simulink model "new_lv_trygenerator_mode1"  (Simulink 7.1)
settings: Solver=ode3  StartTime=0.0  StopTime=1000  FixedStep=0.01  RelTol=1e-3
values from neighbouring files (symbols this model uses):
  Jem = 90    [lv_cankaofile.m]    (also in lv_demofile.m = 97.5; lv_demofile1.m = 97.5; lv_demofile2.m = 97.5; lv_demofile3.m = 97.5)
  Jwt = 9e7    (= 90000000)    [lv_cankaofile.m]    (also in lv_demofile.m = 3275300; lv_demofile1.m = 3275300; lv_demofile2.m = 3275300; lv_demofile3.m = 3275300)
  K = 83    [lv_cankaofile.m]    (also in lv_demofile.m; lv_demofile1.m = 75.76; lv_demofile2.m; lv_demofile3.m = 75.76)
  R = 40    [lv_cankaofile.m]    (also in lv_demofile.m = 38.5; lv_demofile1.m = 38.75; lv_demofile2.m = 38.5; lv_demofile3.m = 38.5)
  ro_air = 1.225    [lv_cankaofile.m]    (also in lv_demofile.m = 1.2236; lv_demofile1.m; lv_demofile2.m = 1.2236; lv_demofile3.m)
libraries: simulink x1, DRlib x1
settings Model: Creator=lv  LastModifiedBy=lv

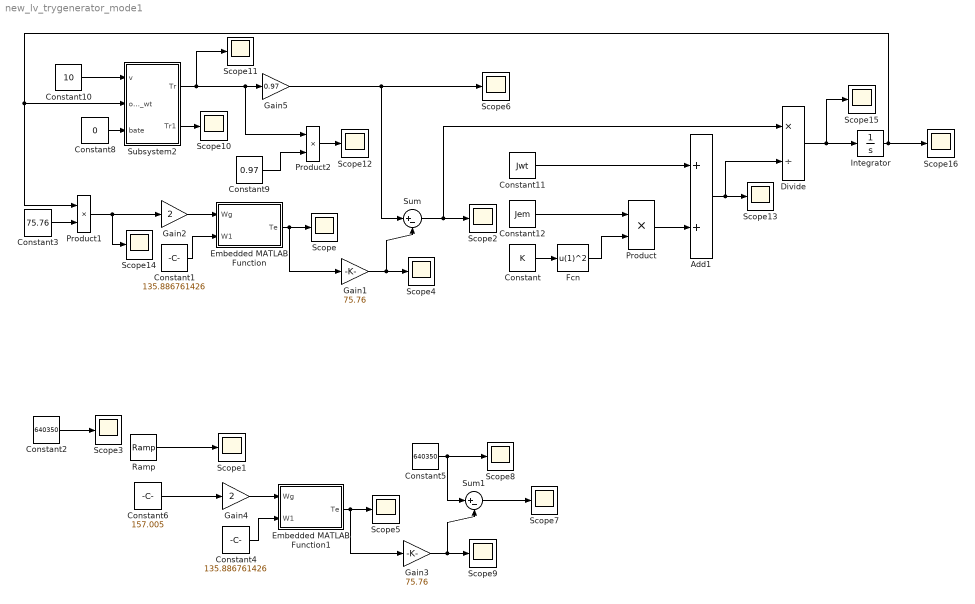
== system new_lv_trygenerator_mode1 ==
  Add1 : Sum  OutDataType=sfix(16)  OutScaling=2^-10
  Constant : Constant  Value=K  OutDataType=sfix(16)  OutScaling=2^0
  Constant1 : Constant  Value=135.886761426  OutDataType=sfix(16)  OutScaling=2^0
  Constant10 : Constant  Value=10  VectorParams1D=off  OutDataType=sfix(16)  OutScaling=2^0
  Constant11 : Constant  Value=Jwt  OutDataType=sfix(16)  OutScaling=2^0
  Constant12 : Constant  Value=Jem  OutDataType=sfix(16)  OutScaling=2^0
  Constant2 : Constant  Value=640350  OutDataType=sfix(16)  OutScaling=2^0
  Constant3 : Constant  Value=75.76  OutDataType=sfix(16)  OutScaling=2^0
  Constant4 : Constant  Value=135.886761426  OutDataType=sfix(16)  OutScaling=2^0
  Constant5 : Constant  Value=640350  OutDataType=sfix(16)  OutScaling=2^0
  Constant6 : Constant  Value=157.005  OutDataType=sfix(16)  OutScaling=2^0
  Constant8 : Constant  Value=0  OutDataType=sfix(16)  OutScaling=2^0
  Constant9 : Constant  Value=0.97  OutDataType=sfix(16)  OutScaling=2^0
  Divide : Product  Inputs=*/  OutDataType=sfix(16)  OutScaling=2^-10
  Embedded MATLAB Function : Stateflow chart
  Embedded MATLAB Function1 : Stateflow chart
  Fcn : Fcn  Expr=u(1)^2
  Gain1 : Gain  Gain=75.76  ParameterDataType=sfix(16)  ParameterScaling=2^0  OutDataType=sfix(16)  OutScaling=2^0
  Gain2 : Gain  Gain=2  ParameterDataType=sfix(16)  ParameterScaling=2^0  OutDataType=sfix(16)  OutScaling=2^0
  Gain3 : Gain  Gain=75.76  ParameterDataType=sfix(16)  ParameterScaling=2^0  OutDataType=sfix(16)  OutScaling=2^0
  Gain4 : Gain  Gain=2  ParameterDataType=sfix(16)  ParameterScaling=2^0  OutDataType=sfix(16)  OutScaling=2^0
  Gain5 : Gain  Gain=0.97  ParameterDataType=sfix(16)  ParameterScaling=2^0  OutDataType=sfix(16)  OutScaling=2^0
  Integrator : Integrator  InitialCondition=2.0724
  Product : Product  OutDataType=sfix(16)  OutScaling=2^0  RndMeth=Zero
  Product1 : Product  OutDataType=sfix(16)  OutScaling=2^0  RndMeth=Zero
  Product2 : Product  OutDataType=sfix(16)  OutScaling=2^0  RndMeth=Zero
  Ramp : simulink/Sources/Ramp  SystemSampleTime=-1  slope=0.05  start=0  X0=157.005
  Scope{,1..16} (17 alike) : Scope
      Scope10 settings: SaveName=ScopeData10
      Scope11 settings: SaveName=ScopeData11
      Scope12 settings: SaveName=ScopeData12
      Scope13 settings: SaveName=ScopeData14
      Scope14 settings: SaveName=ScopeData15
      Scope15 settings: SaveName=ScopeData16
      Scope16 settings: YMin=2.53514  YMax=2.53514  SaveName=ScopeData17
      Scope2 settings: SaveName=ScopeData2
      Scope3 settings: SaveName=ScopeData3
      Scope4 settings: SaveName=ScopeData4
      Scope5 settings: SaveName=ScopeData5
      Scope6 settings: SaveName=ScopeData13
      Scope7 settings: SaveName=ScopeData7
      Scope8 settings: SaveName=ScopeData8
      Scope9 settings: SaveName=ScopeData9
  Subsystem2 : Subsystem
  Sum : Sum  Inputs=|+-  OutDataType=sfix(16)  OutScaling=2^0
  Sum1 : Sum  Inputs=|+-  OutDataType=sfix(16)  OutScaling=2^0
  wires:
  Constant1/1 -> Embedded MATLAB Function/2(W1)
  Embedded MATLAB Function/1(Te) -> Scope/1, Gain1/1
  Gain2/1 -> Embedded MATLAB Function/1(Wg)
  Gain1/1 -> Scope4/1, Sum/2
  Ramp/1 -> Scope1/1
  Sum/1 -> Scope2/1, Divide/1
  Constant4/1 -> Embedded MATLAB Function1/2(W1)
  Embedded MATLAB Function1/1(Te) -> Scope5/1, Gain3/1
  Gain4/1 -> Embedded MATLAB Function1/1(Wg)
  Gain3/1 -> Scope9/1, Sum1/2
  Constant6/1 -> Gain4/1
  Constant5/1 -> Scope8/1, Sum1/1
  Sum1/1 -> Scope7/1
  Constant10/1 -> Subsystem2/1(v)
  Constant8/1 -> Subsystem2/3(bate)
  Subsystem2/1(Tr) -> Scope11/1, Gain5/1, Product2/1
  Subsystem2/2(Tr1) -> Scope10/1
  Gain5/1 -> Scope6/1, Sum/1
  Constant9/1 -> Product2/2
  Product2/1 -> Scope12/1
  Constant2/1 -> Scope3/1
  Fcn/1 -> Product/2
  Constant/1 -> Fcn/1
  Constant12/1 -> Product/1
  Constant11/1 -> Add1/1
  Product/1 -> Add1/2
  Add1/1 -> Scope13/1, Divide/2
  Divide/1 -> Scope15/1, Integrator/1
  Integrator/1 -> Subsystem2/2(omg_wt), Product1/1, Scope16/1
  Product1/1 -> Gain2/1, Scope14/1
  Constant3/1 -> Product1/2

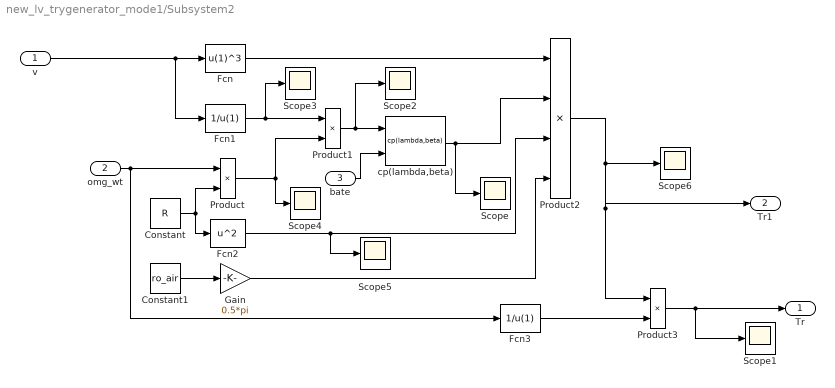
== system new_lv_trygenerator_mode1/Subsystem2 ==
  v : Inport  OutDataType=sfix(16)  OutScaling=2^0
  omg_wt : Inport  Port=2  OutDataType=sfix(16)  OutScaling=2^0
  bate : Inport  Port=3  OutDataType=sfix(16)  OutScaling=2^0
  Constant : Constant  Value=R  OutDataType=sfix(16)  OutScaling=2^0
  Constant1 : Constant  Value=ro_air  OutDataType=sfix(16)  OutScaling=2^0
  Fcn : Fcn  Expr=u(1)^3
  Fcn1 : Fcn  Expr=1/u(1)
  Fcn2 : Fcn  Expr=u^2
  Fcn3 : Fcn  Expr=1/u(1)
  Gain : Gain  Gain=0.5*pi  ParameterDataType=sfix(16)  ParameterScaling=2^0  OutDataType=sfix(16)  OutScaling=2^0
  Product : Product  OutDataType=sfix(16)  OutScaling=2^0  RndMeth=Zero
  Product1 : Product  OutDataType=sfix(16)  OutScaling=2^0  RndMeth=Zero
  Product2 : Product  Inputs=4  OutDataType=sfix(16)  OutScaling=2^0  RndMeth=Zero
  Product3 : Product  OutDataType=sfix(16)  OutScaling=2^0  RndMeth=Zero
  Scope{,1..6} (7 alike) : Scope
      Scope settings: TimeRange=50  YMin=0.1772981595092024  YMax=0.2028981595092024  SaveName=ScopeData4
      Scope1 settings: TimeRange=20  YMin=-1500000  YMax=1500000
      Scope2 settings: SaveName=ScopeData6
      Scope3 settings: SaveName=ScopeData7
      Scope4 settings: SaveName=ScopeData8
      Scope5 settings: YMin=1426.48  YMax=1576.64  SaveName=ScopeData20
      Scope6 settings: TimeRange=20  YMin=-500000  YMax=5e+006  SaveName=ScopeData21
  cp(lambda,beta) : DRlib/Wind Generation/Wind Turbine/cp(lambda,beta)  SystemSampleTime=-1
  Tr : Outport  OutDataType=sfix(16)  OutScaling=2^0
  Tr1 : Outport  Port=2  OutDataType=sfix(16)  OutScaling=2^0
  wires:
  v/1 -> Fcn/1, Fcn1/1
  omg_wt/1 -> Product/1, Fcn3/1
  Constant/1 -> Product/2, Fcn2/1
  Fcn1/1 -> Product1/1, Scope3/1
  Product/1 -> Product1/2, Scope4/1
  Product1/1 -> Scope2/1, cp(lambda,beta)/1
  bate/1 -> cp(lambda,beta)/2
  Fcn/1 -> Product2/1
  cp(lambda,beta)/1 -> Scope/1, Product2/2
  Fcn2/1 -> Product2/3, Scope5/1
  Gain/1 -> Product2/4
  Constant1/1 -> Gain/1
  Product2/1 -> Scope6/1, Product3/1, Tr1/1
  Fcn3/1 -> Product3/2
  Product3/1 -> Scope1/1, Tr/1

== matlab function Embedded MATLAB Function1 ==
  data: Wg input double; Te output double; W1 input double
function Te = fcn(Wg,W1)
%#eml
% This block supports the Embedded MATLAB subset.
% See the help menu for details. 

Te=6855.84/((Wg-W1)*((0.00169-0.813*0.0024*W1/(Wg-W1))^2+(0.03692+0.813*0.03759)^2));
%Te = 6855.84/((Wg-W1)*(0.00169-0.813*0.0024*W1/(Wg-W1))^2+(0.03692+0.813*0.03759)^2);

== matlab function Embedded MATLAB Function ==
  data: Wg input double; Te output double; W1 input double
function Te = fcn(Wg,W1)
%#eml
% This block supports the Embedded MATLAB subset.
% See the help menu for details. 

Te=6855.84/((Wg-W1)*((0.00169-0.813*0.0024*W1/(Wg-W1))^2+(0.03692+0.813*0.03759)^2));
%Te = 6855.84/((Wg-W1)*(0.00169-0.813*0.0024*W1/(Wg-W1))^2+(0.03692+0.813*0.03759)^2);
